simulink model "MCL"  (Simulink 9.0)
settings: Solver=ode45  StartTime=0.0  StopTime=10  RelTol=1e-3  EnableMultiTasking=on
values from neighbouring files (symbols this model uses):
  Abel = 0.0047    [MCL_init.m]
  cbel = 741.22    [MCL_init.m]
  cpc = 2.15*(10^9)    (= 2150000000)    [MCL_init.m]
  ct = 25e-12    (= 2.5e-11)    [MCL_init.m]
  dbel = 1.8    [MCL_init.m]
  g = 9.81    [MCL_init.m]
  h = 1.3    [MCL_init.m]
  Jgp = 0.293*(10^-3)    (= 0.000293)    [MCL_init.m]
  Kemfvca = 35.14    [MCL_init.m]
  Kgpemf = 72.4*(10^-3)    (= 0.0724)    [MCL_init.m]
  Kvcaemf = 35.14    [MCL_init.m]
  Lgp = 1.44*(10^-3)    (= 0.00144)    [MCL_init.m]
  Lhyd = 14.92e6    (= 14920000)    [MCL_init.m]
  Lvca = 2.9*1.0E-03    (= 0.0029)    [MCL_init.m]
  M32LMIN = 1.0E03*60    (= 60000)    [MCL_init.m]
  mbel = 1.1    [MCL_init.m]
  Mlgp = lgp*(ra^2 - ri^2)    (= 3.625e-06)    [MCL_init.m]
  PA2HG = 1.0/HG2PA    (= 0.00750061685073)    [MCL_init.m]
  RADS2TURNMIN = 60/(2*pi)    (= 9.54929658551)    [MCL_init.m]
  Rbf = 1000000000000    [MCL_init.m]
  Rgp = 0.48    [MCL_init.m]
  rhoB = 1.055E03    (= 1055)    [MCL_init.m]
  Rhyd = 572.46e6    (= 572460000)    [MCL_init.m]
  Rvca = 2.6    [MCL_init.m]
  tr0 = 44.9*(10^-6)    (= 4.49e-05)    [MCL_init.m]
  tr1 = 0.3*(10^-3)    (= 0.0003)    [MCL_init.m]
  V0 = V0comp + V0bel    (= 0.000536592894745)    [MCL_init.m]
  Vgpsv = 1.59*(10^-6)    (= 1.59e-06)    [MCL_init.m]
libraries: commnoisgen2 x5
settings Model: Creator=bahram  LastModifiedBy=lohse
settings DataIOCC: LimitDataPoints=on  SignalLoggingSaveFormat=ModelDataLogs
settings OptimizationCC: ExpressionDepthLimit=2147483647
settings DebuggingCC: SolverPrmCheckMsg=warning  MultiTaskDSMMsg=warning  MultiTaskCondExecSysMsg=none  StateNameClashWarn=warning
settings GRTTargetCC: GeneratePreprocessorConditionals=Disable all
settings ConfigComp: CovSFcnEnable=off

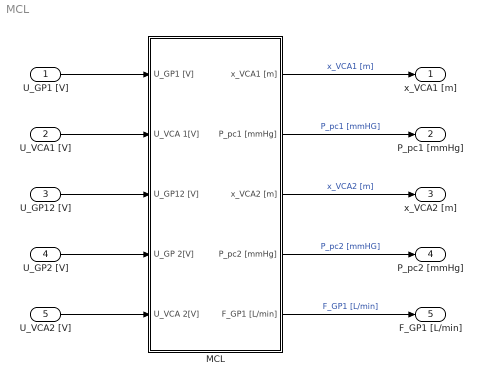
== system MCL ==
  U_GP1 [V] : Inport
  U_VCA1 [V] : Inport  Port=2
  U_GP12 [V] : Inport  Port=3
  U_GP2 [V] : Inport  Port=4
  U_VCA2 [V] : Inport  Port=5
  MCL : Subsystem
  x_VCA1 [m] : Outport
  P_pc1 [mmHg] : Outport  Port=2
  x_VCA2 [m] : Outport  Port=3
  P_pc2 [mmHg] : Outport  Port=4
  F_GP1 [L/min] : Outport  Port=5
  wires:
  MCL/1(x_VCA1 [m]) -> x_VCA1 [m]/1  "x_VCA1 [m]"
  MCL/2(P_pc1 [mmHg]) -> P_pc1 [mmHg]/1  "P_pc1 [mmHG]"
  MCL/3(x_VCA2 [m]) -> x_VCA2 [m]/1  "x_VCA2 [m]"
  MCL/4(P_pc2 [mmHg]) -> P_pc2 [mmHg]/1  "P_pc2 [mmHG]"
  U_GP1 [V]/1 -> MCL/1(U_GP1 [V])
  U_VCA1 [V]/1 -> MCL/2(U_VCA 1[V])
  U_GP12 [V]/1 -> MCL/3(U_GP12 [V])
  U_GP2 [V]/1 -> MCL/4(U_GP 2[V])
  U_VCA2 [V]/1 -> MCL/5(U_VCA 2[V])
  MCL/5(F_GP1 [L/min]) -> F_GP1 [L/min]/1  "F_GP1 [L/min]"

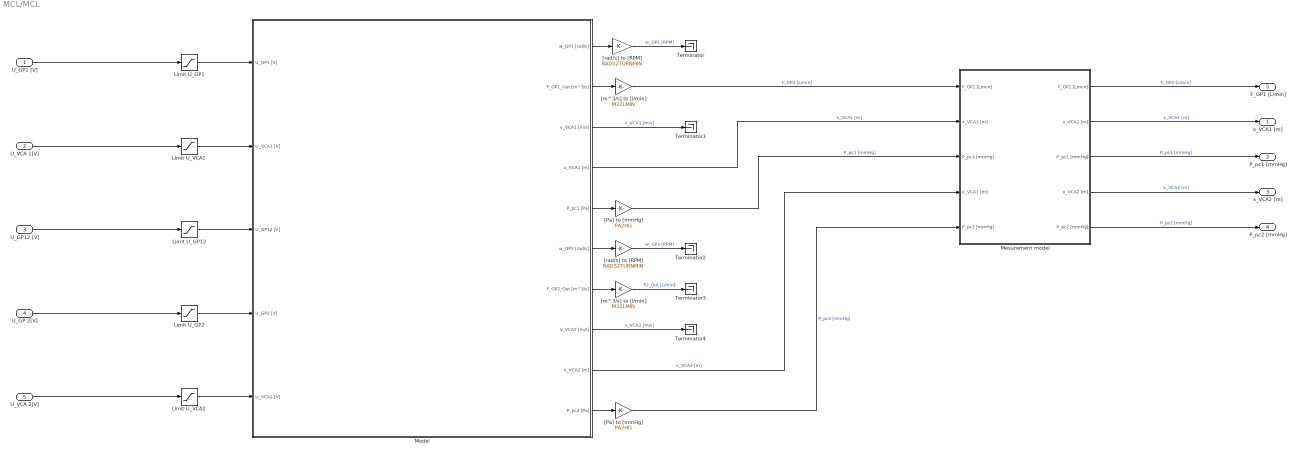
== system MCL/MCL ==
  U_GP1 [V] : Inport
  U_VCA 1[V] : Inport  Port=2
  U_GP12 [V] : Inport  Port=3
  U_GP 2[V] : Inport  Port=4
  U_VCA 2[V] : Inport  Port=5
  Limit U_GP1 : Saturate  UpperLimit=24  LowerLimit=0
  Limit U_GP12 : Saturate  UpperLimit=24  LowerLimit=0
  Limit U_GP2 : Saturate  UpperLimit=24  LowerLimit=0
  Limit U_VCA1 : Saturate  UpperLimit=24  LowerLimit=-24
  Limit U_VCA2 : Saturate  UpperLimit=24  LowerLimit=-24
  Mesurement model : Subsystem
  Model : Subsystem
  Terminator{,1..4} (5 alike) : Terminator
  "[Pa] to [mmHg] " : Gain  Gain=PA2HG
  "[Pa] to [mmHg]  " : Gain  Gain=PA2HG
  "[m^3/s] to [l/min] " : Gain  Gain=M32LMIN
  "[m^3/s] to [l/min]  " : Gain  Gain=M32LMIN
  "[rad/s] to [RPM] " : Gain  Gain=RADS2TURNMIN
  "[rad/s] to [RPM]  " : Gain  Gain=RADS2TURNMIN
  x_VCA1 [m] : Outport
  P_pc1 [mmHg] : Outport  Port=2
  x_VCA2 [m] : Outport  Port=3
  P_pc2 [mmHg] : Outport  Port=4
  F_GP1 [L/min] : Outport  Port=5
  wires:
  Model/1(w_GP1 [rad/s]) -> "[rad/s] to [RPM]  "/1
  Model/2(F_GP1_Out [m^3/s]) -> "[m^3/s] to [l/min]  "/1
  Model/5(P_pc1 [Pa]) -> "[Pa] to [mmHg] "/1
  "[rad/s] to [RPM] "/1 -> Terminator2/1  "w_GP2 [RPM]"
  Model/6(w_GP2 [rad/s]) -> "[rad/s] to [RPM] "/1
  Model/7(F_GP2_Out [m^3/s]) -> "[m^3/s] to [l/min] "/1
  Model/10(P_pc2 [Pa]) -> "[Pa] to [mmHg]  "/1
  "[m^3/s] to [l/min] "/1 -> Terminator3/1  "F2_Out [L/min]"
  Model/8(v_VCA2 [m/s]) -> Terminator4/1  "v_VCA2 [m/s]"
  Model/9(x_VCA2 [m]) -> Mesurement model/4(x_VCA2 [m])  "x_VCA2 [m]"
  "[Pa] to [mmHg]  "/1 -> Mesurement model/5(P_pc2 [mmHg])  "P_pc2 [mmHg]"
  "[rad/s] to [RPM]  "/1 -> Terminator/1  "w_GP1 [RPM]"
  "[m^3/s] to [l/min]  "/1 -> Mesurement model/1(F_GP1 [L/min])  "F_GP1 [L/min]"
  Model/3(v_VCA1 [m/s]) -> Terminator1/1  "v_VCA1 [m/s]"
  Model/4(x_VCA1 [m]) -> Mesurement model/2(x_VCA1 [m])  "x_VCA1 [m]"
  "[Pa] to [mmHg] "/1 -> Mesurement model/3(P_pc1 [mmHg])  "P_pc1 [mmHg]"
  Limit U_GP1/1 -> Model/1(U_GP1 [V])
  Limit U_GP12/1 -> Model/3(U_GP12 [V])
  Limit U_VCA1/1 -> Model/2(U_VCA1 [V])
  Limit U_VCA2/1 -> Model/5(U_VCA2 [V])
  Limit U_GP2/1 -> Model/4(U_GP2 [V])
  Mesurement model/1("F_GP1 [L/min] ") -> F_GP1 [L/min]/1  "F_GP1 [L/min]"
  Mesurement model/2("x_VCA1 [m] ") -> x_VCA1 [m]/1  "x_VCA1 [m]"
  Mesurement model/3("P_pc1 [mmHg] ") -> P_pc1 [mmHg]/1  "P_pc1 [mmHg]"
  Mesurement model/4("x_VCA2 [m] ") -> x_VCA2 [m]/1  "x_VCA2 [m]"
  Mesurement model/5("P_pc2 [mmHg] ") -> P_pc2 [mmHg]/1  "P_pc2 [mmHg]"
  U_GP1 [V]/1 -> Limit U_GP1/1
  U_VCA 1[V]/1 -> Limit U_VCA1/1
  U_GP12 [V]/1 -> Limit U_GP12/1
  U_GP 2[V]/1 -> Limit U_GP2/1
  U_VCA 2[V]/1 -> Limit U_VCA2/1

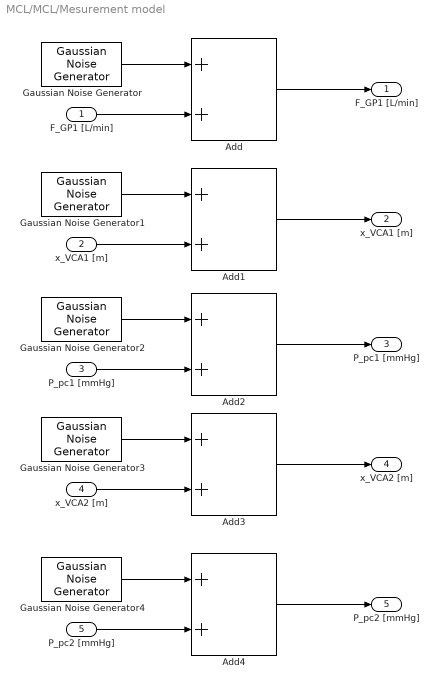
== system MCL/MCL/Mesurement model ==
  F_GP1 [L/min] : Inport
  x_VCA1 [m] : Inport  Port=2
  P_pc1 [mmHg] : Inport  Port=3
  x_VCA2 [m] : Inport  Port=4
  P_pc2 [mmHg] : Inport  Port=5
  Add{,1..4} (5 alike) : Sum
  Gaussian Noise Generator : commnoisgen2/Gaussian Noise Generator  m=0.015  d=0.01  s=100  Ts=0.001  frameBased=off  sampPerFrame=1  orient=off  outDataType=double
  Gaussian Noise Generator1 : commnoisgen2/Gaussian Noise Generator  m=0.0000003  d=0.00000002  s=200  Ts=0.001  frameBased=off  sampPerFrame=1  orient=off  outDataType=double
  Gaussian Noise Generator2 : commnoisgen2/Gaussian Noise Generator  m=0.09  d=0.002  s=115  Ts=0.001  frameBased=off  sampPerFrame=1  orient=off  outDataType=double
  Gaussian Noise Generator3 : commnoisgen2/Gaussian Noise Generator  m=0.0000001  d=0.00000001  s=300  Ts=0.001  frameBased=off  sampPerFrame=1  orient=off  outDataType=double
  Gaussian Noise Generator4 : commnoisgen2/Gaussian Noise Generator  m=0.000002  d=0.0000000015  s=230  Ts=0.001  frameBased=off  sampPerFrame=1  orient=off  outDataType=double
  "F_GP1 [L/min] " : Outport
  "x_VCA1 [m] " : Outport  Port=2
  "P_pc1 [mmHg] " : Outport  Port=3
  "x_VCA2 [m] " : Outport  Port=4
  "P_pc2 [mmHg] " : Outport  Port=5
  wires:
  P_pc1 [mmHg]/1 -> Add2/2
  x_VCA1 [m]/1 -> Add1/2
  P_pc2 [mmHg]/1 -> Add4/2
  x_VCA2 [m]/1 -> Add3/2
  Add1/1 -> "x_VCA1 [m] "/1
  Add2/1 -> "P_pc1 [mmHg] "/1
  Add3/1 -> "x_VCA2 [m] "/1
  Add4/1 -> "P_pc2 [mmHg] "/1
  Add/1 -> "F_GP1 [L/min] "/1
  Gaussian Noise Generator/1 -> Add/1
  F_GP1 [L/min]/1 -> Add/2
  Gaussian Noise Generator1/1 -> Add1/1
  Gaussian Noise Generator2/1 -> Add2/1
  Gaussian Noise Generator3/1 -> Add3/1
  Gaussian Noise Generator4/1 -> Add4/1

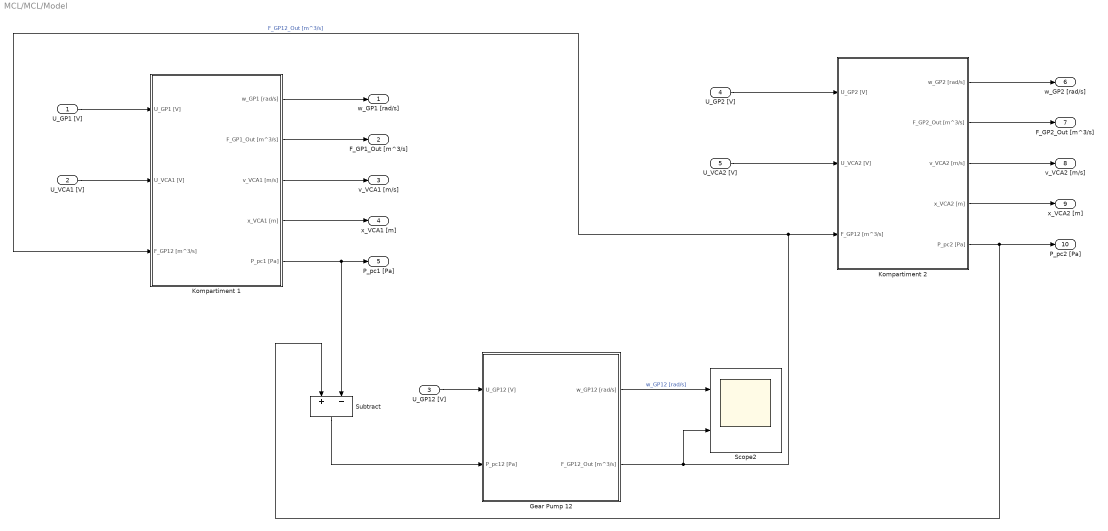
== system MCL/MCL/Model ==
  U_GP1 [V] : Inport
  U_VCA1 [V] : Inport  Port=2
  U_GP12 [V] : Inport  Port=3
  U_GP2 [V] : Inport  Port=4
  U_VCA2 [V] : Inport  Port=5
  Gear Pump 12 : Subsystem
  Kompartiment 1 : Subsystem
  Kompartiment 2 : Subsystem
  Scope2 : Scope  NumInputPorts=2
  Subtract : Sum  Inputs=+-
  w_GP1 [rad/s] : Outport
  F_GP1_Out [m^3/s] : Outport  Port=2
  v_VCA1 [m/s] : Outport  Port=3
  x_VCA1 [m] : Outport  Port=4
  P_pc1 [Pa] : Outport  Port=5
  w_GP2 [rad/s] : Outport  Port=6
  F_GP2_Out [m^3/s] : Outport  Port=7
  v_VCA2 [m/s] : Outport  Port=8
  x_VCA2 [m] : Outport  Port=9
  P_pc2 [Pa] : Outport  Port=10
  wires:
  Gear Pump 12/1(w_GP12 [rad/s]) -> Scope2/1  "w_GP12 [rad/s]"
  Kompartiment 2/1(w_GP2 [rad/s]) -> w_GP2 [rad/s]/1
  Kompartiment 2/2(F_GP2_Out [m^3/s]) -> F_GP2_Out [m^3/s]/1
  Kompartiment 2/4(x_VCA2 [m]) -> x_VCA2 [m]/1
  Kompartiment 2/3("v_VCA2 [m/s]  ") -> v_VCA2 [m/s]/1
  Kompartiment 2/5(P_pc2 [Pa]) -> P_pc2 [Pa]/1, Subtract/1
  Kompartiment 1/3("v_VCA1 [m/s]  ") -> v_VCA1 [m/s]/1
  Kompartiment 1/4(x_VCA1 [m]) -> x_VCA1 [m]/1
  Kompartiment 1/1(w_GP1 [rad/s]) -> w_GP1 [rad/s]/1
  Kompartiment 1/2(F_GP1_Out [m^3/s]) -> F_GP1_Out [m^3/s]/1
  U_GP12 [V]/1 -> Gear Pump 12/1(U_GP12 [V])
  U_GP1 [V]/1 -> Kompartiment 1/1(U_GP1 [V])
  Kompartiment 1/5(P_pc1 [Pa]) -> P_pc1 [Pa]/1, Subtract/2
  U_VCA1 [V]/1 -> Kompartiment 1/2(U_VCA1 [V])
  U_GP2 [V]/1 -> Kompartiment 2/1(U_GP2 [V])
  Subtract/1 -> Gear Pump 12/2(P_pc12 [Pa])
  U_VCA2 [V]/1 -> Kompartiment 2/2(U_VCA2 [V])
  Gear Pump 12/2(F_GP12_Out [m^3/s]) -> Scope2/2, Kompartiment 2/3(F_GP12 [m^3/s]), Kompartiment 1/3(F_GP12 [m^3/s])  "F_GP12_Out [m^3/s]"

== system MCL/MCL/Model/Gear Pump 12 ==
  U_GP12 [V] : Inport
  P_pc12 [Pa] : Inport  Port=2
  Gear Pump 12 ------> w_GP12 & i_GP12 : Subsystem
  Gear Pump 12 -----> F_GP12_Out : Subsystem
  w_GP12 [rad/s] : Outport
  F_GP12_Out [m^3/s] : Outport  Port=2
  wires:
  P_pc12 [Pa]/1 -> Gear Pump 12 -----> F_GP12_Out/2(P_pc12 [PA]), Gear Pump 12 ------> w_GP12 & i_GP12/2(P_pc12 [Pa])
  U_GP12 [V]/1 -> Gear Pump 12 ------> w_GP12 & i_GP12/1(U_GP12 [V])
  Gear Pump 12 ------> w_GP12 & i_GP12/1(w_GP12 [rad/s]) -> Gear Pump 12 -----> F_GP12_Out/1(w_GP12 [rad/s]), w_GP12 [rad/s]/1
  Gear Pump 12 -----> F_GP12_Out/1(F_GP12_Out [m^3/s]) -> F_GP12_Out [m^3/s]/1

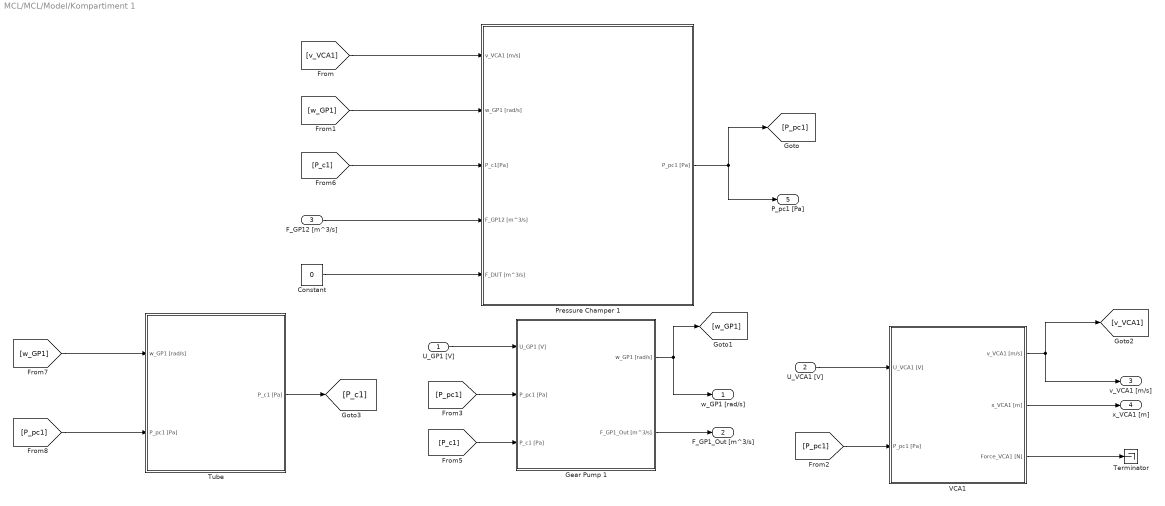
== system MCL/MCL/Model/Kompartiment 1 ==
  U_GP1 [V] : Inport
  U_VCA1 [V] : Inport  Port=2
  F_GP12 [m^3/s] : Inport  Port=3
  Constant : Constant  Value=0
  Gear Pump 1 : Subsystem
  Pressure Champer 1 : Subsystem
  Terminator : Terminator
  Tube : Subsystem
  VCA1 : Subsystem
  w_GP1 [rad/s] : Outport
  F_GP1_Out [m^3/s] : Outport  Port=2
  "v_VCA1 [m/s]  " : Outport  Port=3
  x_VCA1 [m] : Outport  Port=4
  P_pc1 [Pa] : Outport  Port=5
  wires:
  [w_GP1] -> Pressure Champer 1/2(w_GP1 [rad/s])
  U_VCA1 [V]/1 -> VCA1/1(U_VCA1 [V])
  VCA1/2(x_VCA1 [m]) -> x_VCA1 [m]/1
  VCA1/1("v_VCA1 [m/s]  ") -> "v_VCA1 [m/s]  "/1, [v_VCA1]
  Gear Pump 1/2(F_GP1_Out [m^3/s]) -> F_GP1_Out [m^3/s]/1
  Gear Pump 1/1(w_GP1 [rad/s]) -> [w_GP1], w_GP1 [rad/s]/1
  U_GP1 [V]/1 -> Gear Pump 1/1(U_GP1 [V])
  F_GP12 [m^3/s]/1 -> Pressure Champer 1/4(F_GP12 [m^3/s])
  [P_pc1] -> Gear Pump 1/2(P_pc1 [Pa])
  [v_VCA1] -> Pressure Champer 1/1(v_VCA1 [m/s])
  [P_pc1] -> Tube/2(P_pc1 [Pa])
  Tube/1(P_c1 [Pa]) -> [P_c1]
  [P_c1] -> Gear Pump 1/3(P_c1 [Pa])
  [w_GP1] -> Tube/1(w_GP1 [rad/s])
  [P_c1] -> Pressure Champer 1/3(P_c1[Pa])
  [P_pc1] -> VCA1/2("P_pc1 [Pa] ")
  Pressure Champer 1/1(P_pc1 [Pa]) -> [P_pc1], P_pc1 [Pa]/1
  Constant/1 -> Pressure Champer 1/5(F_DUT [m^3/s])
  VCA1/3(Force_VCA1 [N]) -> Terminator/1

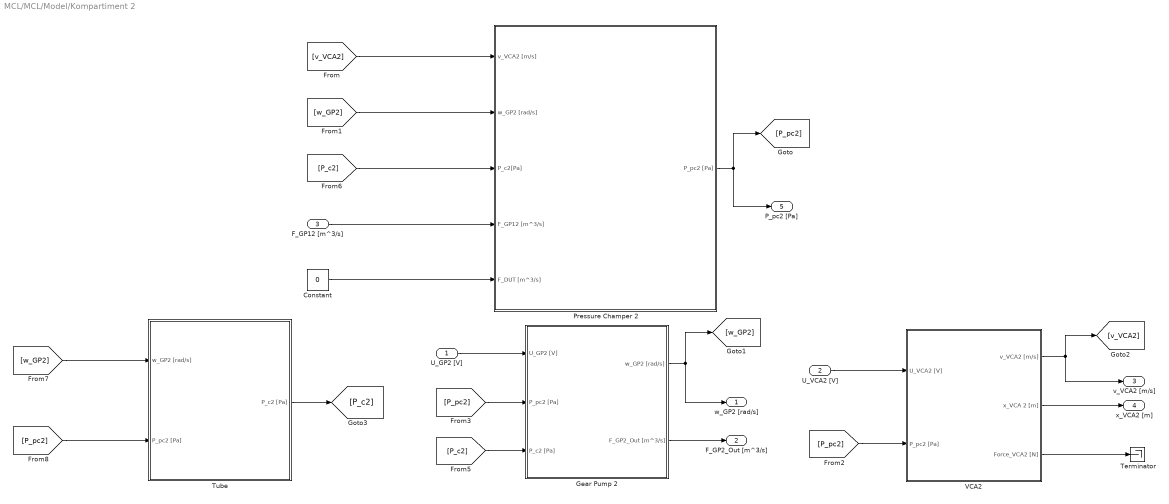
== system MCL/MCL/Model/Kompartiment 2 ==
  U_GP2 [V] : Inport
  U_VCA2 [V] : Inport  Port=2
  F_GP12 [m^3/s] : Inport  Port=3
  Constant : Constant  Value=0
  Gear Pump 2 : Subsystem
  Pressure Champer 2 : Subsystem
  Terminator : Terminator
  Tube : Subsystem
  VCA2 : Subsystem
  w_GP2 [rad/s] : Outport
  F_GP2_Out [m^3/s] : Outport  Port=2
  "v_VCA2 [m/s]  " : Outport  Port=3
  x_VCA2 [m] : Outport  Port=4
  P_pc2 [Pa] : Outport  Port=5
  wires:
  [w_GP2] -> Pressure Champer 2/2(w_GP2 [rad/s])
  U_VCA2 [V]/1 -> VCA2/1(U_VCA2 [V])
  VCA2/2(x_VCA 2 [m]) -> x_VCA2 [m]/1
  VCA2/1("v_VCA2 [m/s]  ") -> "v_VCA2 [m/s]  "/1, [v_VCA2]
  Gear Pump 2/2(F_GP2_Out [m^3/s]) -> F_GP2_Out [m^3/s]/1
  Gear Pump 2/1(w_GP2 [rad/s]) -> [w_GP2], w_GP2 [rad/s]/1
  U_GP2 [V]/1 -> Gear Pump 2/1(U_GP2 [V])
  F_GP12 [m^3/s]/1 -> Pressure Champer 2/4(F_GP12 [m^3/s])
  [P_pc2] -> Gear Pump 2/2(P_pc2 [Pa])
  [v_VCA2] -> Pressure Champer 2/1(v_VCA2 [m/s])
  [P_pc2] -> Tube/2(P_pc2 [Pa])
  Tube/1(P_c2 [Pa]) -> [P_c2]
  [P_c2] -> Gear Pump 2/3(P_c2 [Pa])
  [w_GP2] -> Tube/1(w_GP2 [rad/s])
  [P_c2] -> Pressure Champer 2/3(P_c2[Pa])
  [P_pc2] -> VCA2/2("P_pc2 [Pa] ")
  Pressure Champer 2/1(P_pc2 [Pa]) -> P_pc2 [Pa]/1, [P_pc2]
  Constant/1 -> Pressure Champer 2/5(F_DUT [m^3/s])
  VCA2/3(Force_VCA2 [N]) -> Terminator/1

== system MCL/MCL/Model/Gear Pump 12/Gear Pump 12 ------> w_GP12 & i_GP12 ==
  U_GP12 [V] : Inport
  P_pc12 [Pa] : Inport  Port=2
  Gear Pump_12 ----> i_GP12 : Subsystem
  Gear Pump_12 ----> w_GP12 : Subsystem
  Limit i_GP12 : Saturate  UpperLimit=7.5  LowerLimit=-7.5
  w_GP12 [rad/s] : Outport
  wires:
  P_pc12 [Pa]/1 -> Gear Pump_12 ----> w_GP12/2(P_pc12 [Pa])
  Gear Pump_12 ----> w_GP12/1(w_GP12 [rad/s]) -> w_GP12 [rad/s]/1, Gear Pump_12 ----> i_GP12/1(w_GP12 [rad/s])
  U_GP12 [V]/1 -> Gear Pump_12 ----> i_GP12/3(U_GP12 [V])
  Gear Pump_12 ----> i_GP12/1(i_GP12 [A]) -> Limit i_GP12/1
  Limit i_GP12/1 -> Gear Pump_12 ----> w_GP12/1(i_GP12 [A]), Gear Pump_12 ----> i_GP12/2("i_GP12 [A] ")

== system MCL/MCL/Model/Gear Pump 12/Gear Pump 12 -----> F_GP12_Out ==
  w_GP12 [rad/s] : Inport
  P_pc12 [PA] : Inport  Port=2
  Divide : Product  Inputs=*/
  Product : Product  RndMeth=Zero
  Rbf [Pa/(m^3/s)] : Constant  Value=Rbf
  Subtract1 : Sum  Inputs=+-
  Vgpsv [m^3] : Constant  Value=Vgpsv
  F_GP12_Out [m^3/s] : Outport
  wires:
  Vgpsv [m^3]/1 -> Product/2
  Subtract1/1 -> F_GP12_Out [m^3/s]/1
  P_pc12 [PA]/1 -> Divide/1
  w_GP12 [rad/s]/1 -> Product/1
  Rbf [Pa/(m^3/s)]/1 -> Divide/2
  Product/1 -> Subtract1/1
  Divide/1 -> Subtract1/2

== system MCL/MCL/Model/Kompartiment 1/Gear Pump 1 ==
  U_GP1 [V] : Inport
  P_pc1 [Pa] : Inport  Port=2
  P_c1 [Pa] : Inport  Port=3
  Gear Pump 1 ------> w_GP1 & i_GP1 : Subsystem
  Gear Pump 1 -----> F_GP1_Out : Subsystem
  w_GP1 [rad/s] : Outport
  F_GP1_Out [m^3/s] : Outport  Port=2
  wires:
  P_pc1 [Pa]/1 -> Gear Pump 1 -----> F_GP1_Out/2(P_pc1 [Pa]), Gear Pump 1 ------> w_GP1 & i_GP1/2(P_pc1 [Pa])
  U_GP1 [V]/1 -> Gear Pump 1 ------> w_GP1 & i_GP1/1(U_GP1 [V])
  P_c1 [Pa]/1 -> Gear Pump 1 -----> F_GP1_Out/3(P_c1 [Pa]), Gear Pump 1 ------> w_GP1 & i_GP1/3(P_c1 [Pa])
  Gear Pump 1 ------> w_GP1 & i_GP1/1(w_GP1 [rad/s]) -> w_GP1 [rad/s]/1, Gear Pump 1 -----> F_GP1_Out/1(w_GP1 [rad/s])
  Gear Pump 1 -----> F_GP1_Out/1(F_GP1_Out [m^3/s]) -> F_GP1_Out [m^3/s]/1

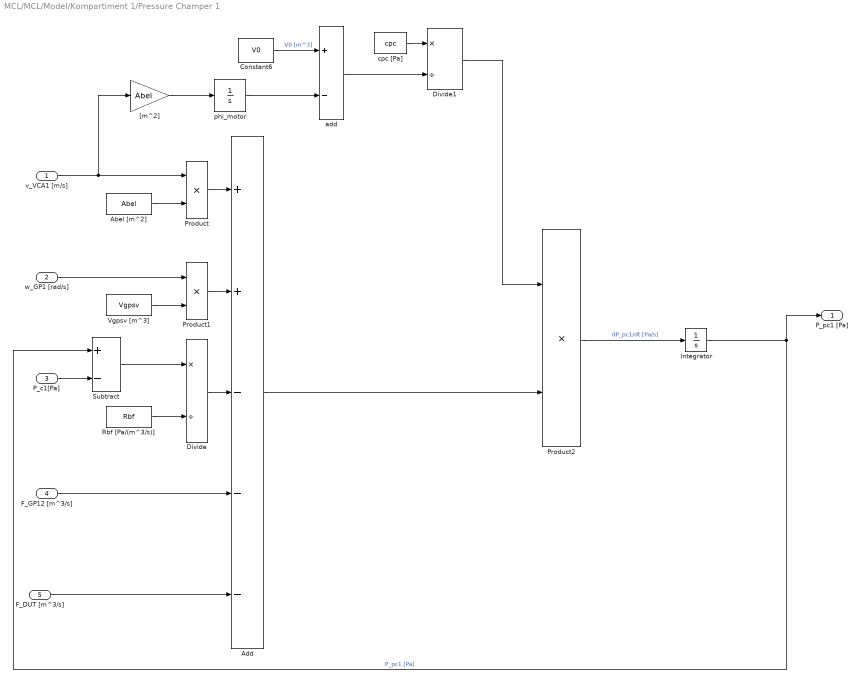
== system MCL/MCL/Model/Kompartiment 1/Pressure Champer 1 ==
  v_VCA1 [m/s] : Inport
  w_GP1 [rad/s] : Inport  Port=2
  P_c1[Pa] : Inport  Port=3
  F_GP12 [m^3/s] : Inport  Port=4
  F_DUT [m^3/s] : Inport  Port=5
  Abel [m^2] : Constant  Value=Abel
  Add : Sum  Inputs=++---
  Constant6 : Constant  Value=V0
  Divide : Product  Inputs=*/
  Divide1 : Product  Inputs=*/
  Integrator : Integrator
  Product : Product  RndMeth=Zero
  Product1 : Product  RndMeth=Zero
  Product2 : Product  RndMeth=Zero
  Rbf [Pa/(m^3/s)] : Constant  Value=Rbf
  Subtract : Sum  Inputs=+-
  Vgpsv [m^3] : Constant  Value=Vgpsv
  "[m^2]" : Gain  Gain=Abel
  add : Sum  Inputs=+-
  cpc [Pa] : Constant  Value=cpc
  phi_motor : Integrator
  P_pc1 [Pa] : Outport
  wires:
  Abel [m^2]/1 -> Product/2
  Subtract/1 -> Divide/1
  P_c1[Pa]/1 -> Subtract/2
  Rbf [Pa/(m^3/s)]/1 -> Divide/2
  Product1/1 -> Add/2
  Product/1 -> Add/1
  Divide/1 -> Add/3
  F_GP12 [m^3/s]/1 -> Add/4
  cpc [Pa]/1 -> Divide1/1
  Divide1/1 -> Product2/1
  Vgpsv [m^3]/1 -> Product1/2
  w_GP1 [rad/s]/1 -> Product1/1
  v_VCA1 [m/s]/1 -> "[m^2]"/1, Product/1
  Integrator/1 -> P_pc1 [Pa]/1, Subtract/1  "P_pc1 [Pa]"
  Add/1 -> Product2/2
  Constant6/1 -> add/1  "V0 [m^3]"
  "[m^2]"/1 -> phi_motor/1
  add/1 -> Divide1/2
  phi_motor/1 -> add/2
  Product2/1 -> Integrator/1  "dP_pc1/dt [Pa/s]"
  F_DUT [m^3/s]/1 -> Add/5

== system MCL/MCL/Model/Kompartiment 1/Tube ==
  w_GP1 [rad/s] : Inport
  P_pc1 [Pa] : Inport  Port=2
  Tube ----> F_hydr1 : Subsystem
  Tube ----> P_c1 : Subsystem
  P_c1 [Pa] : Outport
  wires:
  w_GP1 [rad/s]/1 -> Tube ----> P_c1/2(w_GP1 [rad/s])
  P_pc1 [Pa]/1 -> Tube ----> P_c1/3(P_pc1 [Pa])
  Tube ----> F_hydr1/1(F_hydr1 [m^3/s]) -> Tube ----> P_c1/1(F_hydr1 [m^3/s])
  Tube ----> P_c1/1(P_c1 [Pa]) -> P_c1 [Pa]/1, Tube ----> F_hydr1/1(" P_c1 [Pa] ")

== system MCL/MCL/Model/Kompartiment 1/VCA1 ==
  U_VCA1 [V] : Inport
  "P_pc1 [Pa] " : Inport  Port=2
  Force(X_VCA) / I_VCA [N/A] : Fcn  Expr=(-6.308*10^4)*u^2+(4.33*10^(-14))*u+35.2
  Limit i_VCA1 : Saturate  UpperLimit=7.5  LowerLimit=-7.5
  Limit x_VCA1 : Saturate  UpperLimit=0.0127  LowerLimit=-0.0127
  MATLAB Function : MATLAB Function  TreatAsAtomicUnit=on
  Product : Product  RndMeth=Zero
  Product4 : Product  RndMeth=Zero
  VCA 1-----> v_VCA1 & x_VCA1 : Subsystem
  VCA1 -----> i_VCA1 : Subsystem
  "v_VCA1 [m/s]  " : Outport
  x_VCA1 [m] : Outport  Port=2
  Force_VCA1 [N] : Outport  Port=3
  wires:
  VCA 1-----> v_VCA1 & x_VCA1/1("v_VCA1 [m/s]  ") -> Product/1, VCA1 -----> i_VCA1/2(v_VCA1 [m/s]), VCA 1-----> v_VCA1 & x_VCA1/3("v_VCA1 [m/s] ")
  VCA1 -----> i_VCA1/1("i_VCA1 [A] ") -> Limit i_VCA1/1  "i_VCA1 [A]"
  U_VCA1 [V]/1 -> VCA1 -----> i_VCA1/3(U_VCA1 [V])
  "P_pc1 [Pa] "/1 -> VCA 1-----> v_VCA1 & x_VCA1/4("P_pc1 [Pa] ")
  VCA 1-----> v_VCA1 & x_VCA1/2(x_VCA 1 [m]) -> Limit x_VCA1/1
  Limit i_VCA1/1 -> VCA1 -----> i_VCA1/1(i_VCA1 [A]), VCA 1-----> v_VCA1 & x_VCA1/1(i_VCA1 [A]), Product4/2
  Limit x_VCA1/1 -> x_VCA1 [m]/1, MATLAB Function/1(u), Force(X_VCA) / I_VCA [N/A]/1, VCA 1-----> v_VCA1 & x_VCA1/2(x_VCA1 [m])
  Force(X_VCA) / I_VCA [N/A]/1 -> Product4/1
  Product4/1 -> Force_VCA1 [N]/1  "Force_VCA1 [N]"
  MATLAB Function/1(y) -> Product/2
  Product/1 -> "v_VCA1 [m/s]  "/1

== system MCL/MCL/Model/Kompartiment 2/Gear Pump 2 ==
  U_GP2 [V] : Inport
  P_pc2 [Pa] : Inport  Port=2
  P_c2 [Pa] : Inport  Port=3
  Gear Pump 2 ------> w_GP2 & i_GP2 : Subsystem
  Gear Pump 2 -----> F_GP2_Out : Subsystem
  w_GP2 [rad/s] : Outport
  F_GP2_Out [m^3/s] : Outport  Port=2
  wires:
  P_pc2 [Pa]/1 -> Gear Pump 2 -----> F_GP2_Out/2(P_pc2 [Pa]), Gear Pump 2 ------> w_GP2 & i_GP2/2(P_pc2 [Pa])
  U_GP2 [V]/1 -> Gear Pump 2 ------> w_GP2 & i_GP2/1(U_GP2 [V])
  P_c2 [Pa]/1 -> Gear Pump 2 -----> F_GP2_Out/3(P_c2 [Pa]), Gear Pump 2 ------> w_GP2 & i_GP2/3(P_c2 [Pa])
  Gear Pump 2 ------> w_GP2 & i_GP2/1(w_GP2 [rad/s]) -> w_GP2 [rad/s]/1, Gear Pump 2 -----> F_GP2_Out/1(w_GP2 [rad/s])
  Gear Pump 2 -----> F_GP2_Out/1(F_GP2_Out [m^3/s]) -> F_GP2_Out [m^3/s]/1

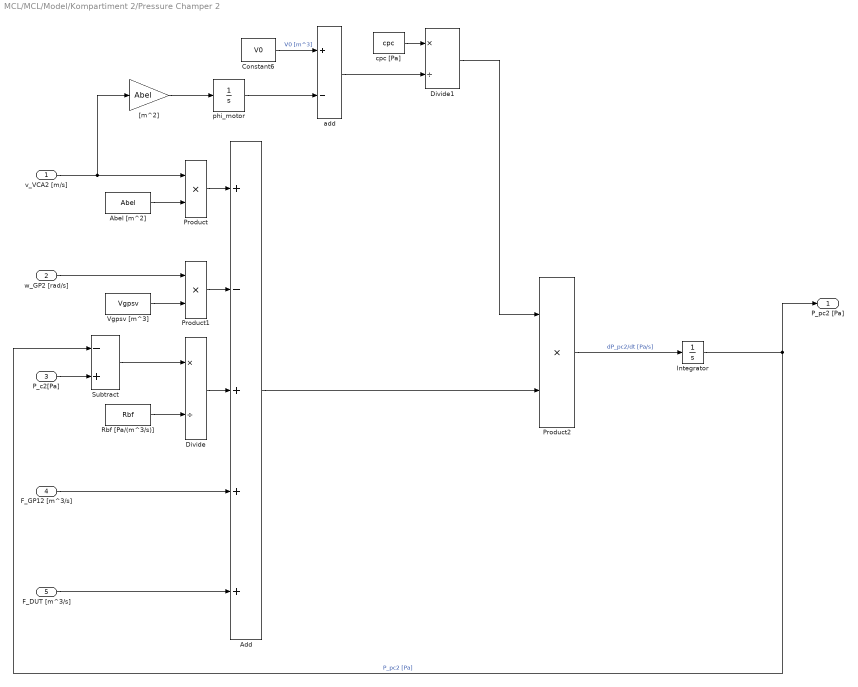
== system MCL/MCL/Model/Kompartiment 2/Pressure Champer 2 ==
  v_VCA2 [m/s] : Inport
  w_GP2 [rad/s] : Inport  Port=2
  P_c2[Pa] : Inport  Port=3
  F_GP12 [m^3/s] : Inport  Port=4
  F_DUT [m^3/s] : Inport  Port=5
  Abel [m^2] : Constant  Value=Abel
  Add : Sum  Inputs=+-+++
  Constant6 : Constant  Value=V0
  Divide : Product  Inputs=*/
  Divide1 : Product  Inputs=*/
  Integrator : Integrator
  Product : Product  RndMeth=Zero
  Product1 : Product  RndMeth=Zero
  Product2 : Product  RndMeth=Zero
  Rbf [Pa/(m^3/s)] : Constant  Value=Rbf
  Subtract : Sum  Inputs=-+
  Vgpsv [m^3] : Constant  Value=Vgpsv
  "[m^2]" : Gain  Gain=Abel
  add : Sum  Inputs=+-
  cpc [Pa] : Constant  Value=cpc
  phi_motor : Integrator
  P_pc2 [Pa] : Outport
  wires:
  Abel [m^2]/1 -> Product/2
  Subtract/1 -> Divide/1
  P_c2[Pa]/1 -> Subtract/2
  Rbf [Pa/(m^3/s)]/1 -> Divide/2
  Product1/1 -> Add/2
  Product/1 -> Add/1
  Divide/1 -> Add/3
  F_GP12 [m^3/s]/1 -> Add/4
  cpc [Pa]/1 -> Divide1/1
  Divide1/1 -> Product2/1
  Vgpsv [m^3]/1 -> Product1/2
  w_GP2 [rad/s]/1 -> Product1/1
  v_VCA2 [m/s]/1 -> "[m^2]"/1, Product/1
  Integrator/1 -> P_pc2 [Pa]/1, Subtract/1  "P_pc2 [Pa]"
  Add/1 -> Product2/2
  Constant6/1 -> add/1  "V0 [m^3]"
  "[m^2]"/1 -> phi_motor/1
  add/1 -> Divide1/2
  phi_motor/1 -> add/2
  Product2/1 -> Integrator/1  "dP_pc2/dt [Pa/s]"
  F_DUT [m^3/s]/1 -> Add/5

== system MCL/MCL/Model/Kompartiment 2/Tube ==
  w_GP2 [rad/s] : Inport
  P_pc2 [Pa] : Inport  Port=2
  Tube ----> F_hydr2 : Subsystem
  Tube ----> P_c2 : Subsystem
  P_c2 [Pa] : Outport
  wires:
  w_GP2 [rad/s]/1 -> Tube ----> P_c2/2(w_GP2 [rad/s])
  P_pc2 [Pa]/1 -> Tube ----> P_c2/3(P_pc2 [Pa])
  Tube ----> F_hydr2/1(F_hydr2 [m^3/s]) -> Tube ----> P_c2/1(F_hydr2 [m^3/s])
  Tube ----> P_c2/1(P_c2 [Pa]) -> P_c2 [Pa]/1, Tube ----> F_hydr2/1(" P_c2 [Pa] ")

== system MCL/MCL/Model/Kompartiment 2/VCA2 ==
  U_VCA2 [V] : Inport
  "P_pc2 [Pa] " : Inport  Port=2
  Force(X_VCA) / I_VCA [N/A] : Fcn  Expr=(-6.308*10^4)*u^2+(4.33*10^(-14))*u+35.2
  Limit i_VCA2 : Saturate  UpperLimit=7.5  LowerLimit=-7.5
  Limit x_VCA2 : Saturate  UpperLimit=0.0127  LowerLimit=-0.0127
  MATLAB Function1 : MATLAB Function  TreatAsAtomicUnit=on
  Product1 : Product  RndMeth=Zero
  Product4 : Product  RndMeth=Zero
  VCA 2-----> v_VCA2 & x_VCA2 : Subsystem
  VCA2 -----> i_VCA2 : Subsystem
  "v_VCA2 [m/s]  " : Outport
  x_VCA 2 [m] : Outport  Port=2
  Force_VCA2 [N] : Outport  Port=3
  wires:
  VCA 2-----> v_VCA2 & x_VCA2/1("v_VCA2 [m/s]  ") -> Product1/1, VCA2 -----> i_VCA2/2(v_VCA2 [m/s]), VCA 2-----> v_VCA2 & x_VCA2/3("v_VCA2 [m/s] ")
  VCA2 -----> i_VCA2/1("i_VCA2 [A] ") -> Limit i_VCA2/1  "i_VCA2 [A]"
  U_VCA2 [V]/1 -> VCA2 -----> i_VCA2/3(U_VCA2 [V])
  "P_pc2 [Pa] "/1 -> VCA 2-----> v_VCA2 & x_VCA2/4("P_pc2 [Pa] ")
  VCA 2-----> v_VCA2 & x_VCA2/2(x_VCA 2 [m]) -> Limit x_VCA2/1
  Limit i_VCA2/1 -> VCA2 -----> i_VCA2/1(i_VCA2 [A]), VCA 2-----> v_VCA2 & x_VCA2/1(i_VCA2 [A]), Product4/2
  Limit x_VCA2/1 -> MATLAB Function1/1(u), x_VCA 2 [m]/1, Force(X_VCA) / I_VCA [N/A]/1, VCA 2-----> v_VCA2 & x_VCA2/2(x_VCA2 [m])
  Force(X_VCA) / I_VCA [N/A]/1 -> Product4/1
  Product4/1 -> Force_VCA2 [N]/1  "Force_VCA2 [N]"
  MATLAB Function1/1(y) -> Product1/2
  Product1/1 -> "v_VCA2 [m/s]  "/1

== system MCL/MCL/Model/Gear Pump 12/Gear Pump 12 ------> w_GP12 & i_GP12/Gear Pump_12 ----> i_GP12 ==
  w_GP12 [rad/s] : Inport
  "i_GP12 [A] " : Inport  Port=2
  U_GP12 [V] : Inport  Port=3
  Add : Sum  Inputs=--+
  Divide : Product  Inputs=*/
  Integrator : Integrator
  Kgpemf [Vs] : Constant  Value=Kgpemf
  Lgp [H] : Constant  Value=Lgp
  Product : Product  RndMeth=Zero
  Product1 : Product  RndMeth=Zero
  Rgp [Ohm] : Constant  Value=Rgp
  i_GP12 [A] : Outport
  wires:
  w_GP12 [rad/s]/1 -> Product/1
  Kgpemf [Vs]/1 -> Product/2
  "i_GP12 [A] "/1 -> Product1/1
  Rgp [Ohm]/1 -> Product1/2
  Product1/1 -> Add/2
  Product/1 -> Add/1
  U_GP12 [V]/1 -> Add/3
  Lgp [H]/1 -> Divide/2
  Divide/1 -> Integrator/1  "di_GP12/dt [A/s]"
  Add/1 -> Divide/1
  Integrator/1 -> i_GP12 [A]/1  "i_GP12[A]"

== system MCL/MCL/Model/Gear Pump 12/Gear Pump 12 ------> w_GP12 & i_GP12/Gear Pump_12 ----> w_GP12 ==
  i_GP12 [A] : Inport
  P_pc12 [Pa] : Inport  Port=2
  Constant : Constant  Value=tr0
  Constant1 : Constant  Value=tr1
  Divide : Product  Inputs=*/
  Integrator : Integrator
  Kgpemf [Vs] : Constant  Value=Kgpemf
  Mlgp [m^3] : Constant  Value=Mlgp
  Product{,1..3} (4 alike) : Product  RndMeth=Zero
  Sign : Signum  ZeroCross=off
  Subtract1 : Sum  Inputs=+---
  jgp [kgm^2] : Constant  Value=Jgp
  w_GP12 [rad/s] : Outport
  wires:
  Subtract1/1 -> Divide/1
  jgp [kgm^2]/1 -> Divide/2
  Integrator/1 -> Product3/1, Sign/1, w_GP12 [rad/s]/1  "w_GP12[rad/s]"
  Divide/1 -> Integrator/1  "dw_GP12/dt [rad/s^2]"
  i_GP12 [A]/1 -> Product/1
  Kgpemf [Vs]/1 -> Product/2
  Product/1 -> Subtract1/1
  Product1/1 -> Subtract1/2
  P_pc12 [Pa]/1 -> Product1/1
  Mlgp [m^3]/1 -> Product1/2
  Sign/1 -> Product2/1
  Constant/1 -> Product2/2
  Product3/1 -> Subtract1/4
  Constant1/1 -> Product3/2
  Product2/1 -> Subtract1/3

== system MCL/MCL/Model/Kompartiment 1/Gear Pump 1/Gear Pump 1 ------> w_GP1 & i_GP1 ==
  U_GP1 [V] : Inport
  P_pc1 [Pa] : Inport  Port=2
  P_c1 [Pa] : Inport  Port=3
  "Gear Pump_1 ----> i_GP1 " : Subsystem
  Gear Pump_1 ----> w_GP1 : Subsystem
  Limit i_GP1 : Saturate  UpperLimit=7.5  LowerLimit=-7.5
  w_GP1 [rad/s] : Outport
  wires:
  P_c1 [Pa]/1 -> Gear Pump_1 ----> w_GP1/3(P_c1 [Pa])
  P_pc1 [Pa]/1 -> Gear Pump_1 ----> w_GP1/2(P_pc1 [Pa])
  Gear Pump_1 ----> w_GP1/1(w_GP1 [rad/s]) -> w_GP1 [rad/s]/1, "Gear Pump_1 ----> i_GP1 "/1(w_GP1 [rad/s])
  U_GP1 [V]/1 -> "Gear Pump_1 ----> i_GP1 "/3(U_GP1 [V])
  "Gear Pump_1 ----> i_GP1 "/1(i_GP1 [A]) -> Limit i_GP1/1
  Limit i_GP1/1 -> Gear Pump_1 ----> w_GP1/1(i_GP1 [A]), "Gear Pump_1 ----> i_GP1 "/2("i_GP1 [A] ")

== system MCL/MCL/Model/Kompartiment 1/Gear Pump 1/Gear Pump 1 -----> F_GP1_Out ==
  w_GP1 [rad/s] : Inport
  P_pc1 [Pa] : Inport  Port=2
  P_c1 [Pa] : Inport  Port=3
  Divide : Product  Inputs=*/
  Product : Product  RndMeth=Zero
  Rbf [Pa/(m^3/s)] : Constant  Value=Rbf
  Subtract : Sum  Inputs=+-
  Subtract1 : Sum  Inputs=+-
  Vgpsv [m^3] : Constant  Value=Vgpsv
  F_GP1_Out [m^3/s] : Outport
  wires:
  Vgpsv [m^3]/1 -> Product/2
  Subtract1/1 -> F_GP1_Out [m^3/s]/1
  Subtract/1 -> Divide/1
  w_GP1 [rad/s]/1 -> Product/1
  P_pc1 [Pa]/1 -> Subtract/1
  P_c1 [Pa]/1 -> Subtract/2
  Rbf [Pa/(m^3/s)]/1 -> Divide/2
  Product/1 -> Subtract1/1
  Divide/1 -> Subtract1/2

== system MCL/MCL/Model/Kompartiment 1/Tube/Tube ----> F_hydr1 ==
  " P_c1 [Pa] " : Inport
  Add : Sum  Inputs=--+
  Divide : Product  Inputs=*/
  Integrator : Integrator
  Lhyd [kg/m^4] : Constant  Value=Lhyd
  Product : Product  RndMeth=Zero
  Rhyd [Pa/(m^3/s)] : Constant  Value=Rhyd
  "[Pa]" : Constant  Value=rhoB*g*h
  F_hydr1 [m^3/s] : Outport
  wires:
  Integrator/1 -> F_hydr1 [m^3/s]/1, Product/1  "F_hydr1 [m^3/s]"
  " P_c1 [Pa] "/1 -> Add/1
  Product/1 -> Add/2
  Lhyd [kg/m^4]/1 -> Divide/2
  Add/1 -> Divide/1
  Divide/1 -> Integrator/1  "dF_hydr1/dt [m^3/s^2]"
  Rhyd [Pa/(m^3/s)]/1 -> Product/2
  "[Pa]"/1 -> Add/3

== system MCL/MCL/Model/Kompartiment 1/Tube/Tube ----> P_c1 ==
  F_hydr1 [m^3/s] : Inport
  w_GP1 [rad/s] : Inport  Port=2
  P_pc1 [Pa] : Inport  Port=3
  Add : Sum  Inputs=+-+
  Divide : Product  Inputs=*/
  Divide1 : Product  Inputs=*/
  Integrator : Integrator
  Product : Product  RndMeth=Zero
  Subtract : Sum  Inputs=+-
  Vgpsv [m^3] : Constant  Value=Vgpsv
  "[Pa/(m^3/s)]" : Constant  Value=Rbf
  ct [s^2*m^4/Kg] : Constant  Value=ct
  P_c1 [Pa] : Outport
  wires:
  Vgpsv [m^3]/1 -> Product/2
  w_GP1 [rad/s]/1 -> Product/1
  Subtract/1 -> Divide/1
  F_hydr1 [m^3/s]/1 -> Add/1
  P_pc1 [Pa]/1 -> Subtract/1
  "[Pa/(m^3/s)]"/1 -> Divide/2
  Product/1 -> Add/2
  Divide/1 -> Add/3
  ct [s^2*m^4/Kg]/1 -> Divide1/2
  Add/1 -> Divide1/1
  Integrator/1 -> Subtract/2, P_c1 [Pa]/1  "P_c1 [Pa]"
  Divide1/1 -> Integrator/1  "dP_c1/dt [Pa/s]"

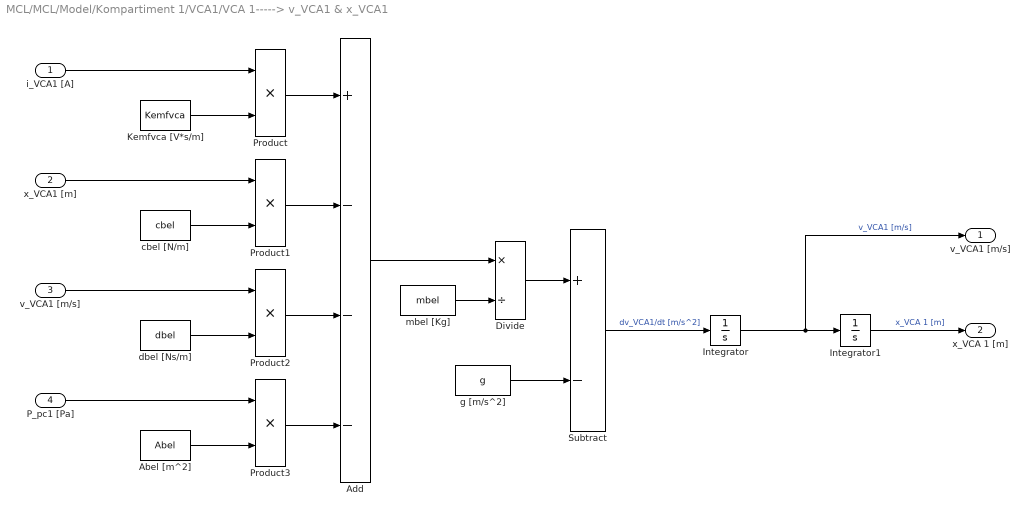
== system MCL/MCL/Model/Kompartiment 1/VCA1/VCA 1-----> v_VCA1 & x_VCA1 ==
  i_VCA1 [A] : Inport
  x_VCA1 [m] : Inport  Port=2
  "v_VCA1 [m/s] " : Inport  Port=3
  "P_pc1 [Pa] " : Inport  Port=4
  Abel [m^2] : Constant  Value=Abel
  Add : Sum  Inputs=+---
  Divide : Product  Inputs=*/
  Integrator : Integrator
  Integrator1 : Integrator
  Kemfvca [V*s/m] : Constant  Value=Kemfvca
  Product{,1..3} (4 alike) : Product  RndMeth=Zero
  Subtract : Sum  Inputs=+-
  cbel [N/m] : Constant  Value=cbel
  dbel [Ns/m] : Constant  Value=dbel
  g [m/s^2] : Constant  Value=g
  mbel [Kg] : Constant  Value=mbel
  "v_VCA1 [m/s]  " : Outport
  x_VCA 1 [m] : Outport  Port=2
  wires:
  Divide/1 -> Subtract/1
  Integrator1/1 -> x_VCA 1 [m]/1  "x_VCA 1 [m]"
  dbel [Ns/m]/1 -> Product2/2
  Kemfvca [V*s/m]/1 -> Product/2
  Add/1 -> Divide/1
  cbel [N/m]/1 -> Product1/2
  Product/1 -> Add/1
  "v_VCA1 [m/s] "/1 -> Product2/1
  i_VCA1 [A]/1 -> Product/1
  x_VCA1 [m]/1 -> Product1/1
  Product1/1 -> Add/2
  Subtract/1 -> Integrator/1  "dv_VCA1/dt [m/s^2]"
  g [m/s^2]/1 -> Subtract/2
  Product2/1 -> Add/3
  Product3/1 -> Add/4
  Abel [m^2]/1 -> Product3/2
  "P_pc1 [Pa] "/1 -> Product3/1
  mbel [Kg]/1 -> Divide/2
  Integrator/1 -> "v_VCA1 [m/s]  "/1, Integrator1/1  "v_VCA1 [m/s]"

== system MCL/MCL/Model/Kompartiment 1/VCA1/VCA1 -----> i_VCA1 ==
  i_VCA1 [A] : Inport
  v_VCA1 [m/s] : Inport  Port=2
  U_VCA1 [V] : Inport  Port=3
  Add : Sum  Inputs=--+
  Divide : Product  Inputs=*/
  Integrator : Integrator
  Kvcaemf [N/A] : Constant  Value=Kvcaemf
  Lvca [H] : Constant  Value=Lvca
  Product : Product  RndMeth=Zero
  Product1 : Product  RndMeth=Zero
  Rvca [Ohm] : Constant  Value=Rvca
  "i_VCA1 [A] " : Outport
  wires:
  Product/1 -> Add/1
  v_VCA1 [m/s]/1 -> Product1/1
  U_VCA1 [V]/1 -> Add/3
  i_VCA1 [A]/1 -> Product/1
  Rvca [Ohm]/1 -> Product/2
  Product1/1 -> Add/2
  Kvcaemf [N/A]/1 -> Product1/2
  Divide/1 -> Integrator/1  "di_VCA1/dt[A/s]"
  Lvca [H]/1 -> Divide/2
  Integrator/1 -> "i_VCA1 [A] "/1  "i_VCA1 [A]"
  Add/1 -> Divide/1

== system MCL/MCL/Model/Kompartiment 2/Gear Pump 2/Gear Pump 2 ------> w_GP2 & i_GP2 ==
  U_GP2 [V] : Inport
  P_pc2 [Pa] : Inport  Port=2
  P_c2 [Pa] : Inport  Port=3
  "Gear Pump 2 ----> i_GP2 " : Subsystem
  Gear Pump 2 ----> w_GP2 : Subsystem
  Limit i_GP2 : Saturate  UpperLimit=7.5  LowerLimit=-7.5
  w_GP2 [rad/s] : Outport
  wires:
  P_c2 [Pa]/1 -> Gear Pump 2 ----> w_GP2/3(P_c2 [Pa])
  P_pc2 [Pa]/1 -> Gear Pump 2 ----> w_GP2/2(P_pc2 [Pa])
  Gear Pump 2 ----> w_GP2/1(w_GP2 [rad/s]) -> w_GP2 [rad/s]/1, "Gear Pump 2 ----> i_GP2 "/1(w_GP2 [rad/s])
  U_GP2 [V]/1 -> "Gear Pump 2 ----> i_GP2 "/3(U_GP2 [V])
  "Gear Pump 2 ----> i_GP2 "/1(i_GP2 [A]) -> Limit i_GP2/1
  Limit i_GP2/1 -> Gear Pump 2 ----> w_GP2/1(i_GP2 [A]), "Gear Pump 2 ----> i_GP2 "/2("i_GP2 [A] ")

== system MCL/MCL/Model/Kompartiment 2/Gear Pump 2/Gear Pump 2 -----> F_GP2_Out ==
  w_GP2 [rad/s] : Inport
  P_pc2 [Pa] : Inport  Port=2
  P_c2 [Pa] : Inport  Port=3
  Divide : Product  Inputs=*/
  Product : Product  RndMeth=Zero
  Rbf [Pa/(m^3/s)] : Constant  Value=Rbf
  Subtract : Sum  Inputs=-+
  Subtract1 : Sum  Inputs=+-
  Vgpsv [m^3] : Constant  Value=Vgpsv
  F_GP2_Out [m^3/s] : Outport
  wires:
  Vgpsv [m^3]/1 -> Product/2
  Subtract1/1 -> F_GP2_Out [m^3/s]/1
  Subtract/1 -> Divide/1
  w_GP2 [rad/s]/1 -> Product/1
  P_pc2 [Pa]/1 -> Subtract/1
  P_c2 [Pa]/1 -> Subtract/2
  Rbf [Pa/(m^3/s)]/1 -> Divide/2
  Product/1 -> Subtract1/1
  Divide/1 -> Subtract1/2

== system MCL/MCL/Model/Kompartiment 2/Tube/Tube ----> F_hydr2 ==
  " P_c2 [Pa] " : Inport
  Add : Sum  Inputs=---
  Divide : Product  Inputs=*/
  Integrator : Integrator
  Lhyd [kg/m^4] : Constant  Value=Lhyd
  Product : Product  RndMeth=Zero
  Rhyd [Pa/(m^3/s)] : Constant  Value=Rhyd
  "[N/m^2]" : Constant  Value=rhoB*g*h
  F_hydr2 [m^3/s] : Outport
  wires:
  Integrator/1 -> F_hydr2 [m^3/s]/1, Product/1  "F_hydr2 [m^3/s]"
  " P_c2 [Pa] "/1 -> Add/1
  Product/1 -> Add/2
  Lhyd [kg/m^4]/1 -> Divide/2
  Add/1 -> Divide/1
  Divide/1 -> Integrator/1  "dF_hydr2/dt [m^3/s^2]"
  Rhyd [Pa/(m^3/s)]/1 -> Product/2
  "[N/m^2]"/1 -> Add/3

== system MCL/MCL/Model/Kompartiment 2/Tube/Tube ----> P_c2 ==
  F_hydr2 [m^3/s] : Inport
  w_GP2 [rad/s] : Inport  Port=2
  P_pc2 [Pa] : Inport  Port=3
  Add : Sum  Inputs=+-+
  Divide : Product  Inputs=*/
  Divide1 : Product  Inputs=*/
  Integrator : Integrator
  Product : Product  RndMeth=Zero
  Subtract : Sum  Inputs=+-
  Vgpsv [m^3] : Constant  Value=Vgpsv
  "[Pa/(m^3/s)]" : Constant  Value=Rbf
  ct [s^2*m^4/Kg] : Constant  Value=ct
  P_c2 [Pa] : Outport
  wires:
  Vgpsv [m^3]/1 -> Product/2
  w_GP2 [rad/s]/1 -> Product/1
  Subtract/1 -> Divide/1
  F_hydr2 [m^3/s]/1 -> Add/1
  P_pc2 [Pa]/1 -> Subtract/1
  "[Pa/(m^3/s)]"/1 -> Divide/2
  Product/1 -> Add/2
  Divide/1 -> Add/3
  ct [s^2*m^4/Kg]/1 -> Divide1/2
  Add/1 -> Divide1/1
  Integrator/1 -> Subtract/2, P_c2 [Pa]/1  "P_c2 [Pa]"
  Divide1/1 -> Integrator/1  "dP_c2/dt [Pa/s]"

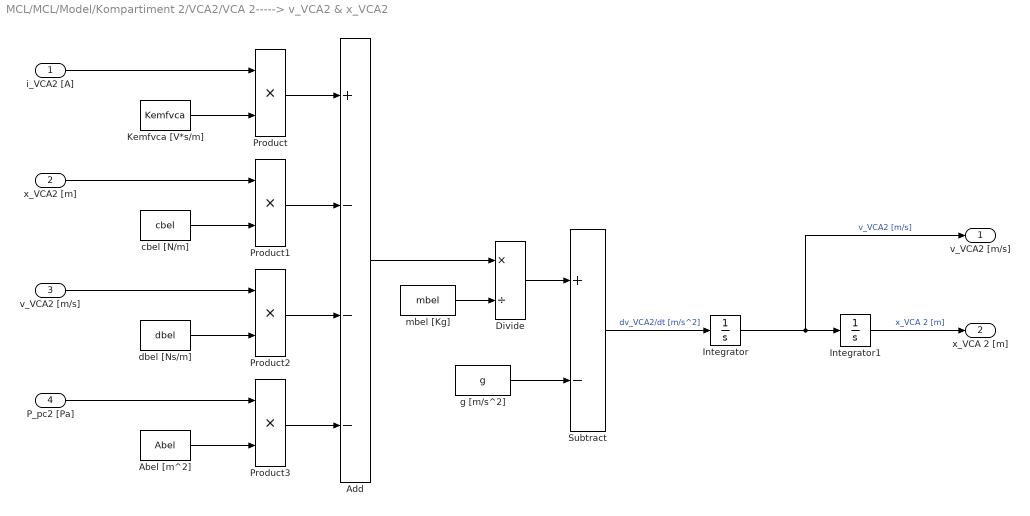
== system MCL/MCL/Model/Kompartiment 2/VCA2/VCA 2-----> v_VCA2 & x_VCA2 ==
  i_VCA2 [A] : Inport
  x_VCA2 [m] : Inport  Port=2
  "v_VCA2 [m/s] " : Inport  Port=3
  "P_pc2 [Pa] " : Inport  Port=4
  Abel [m^2] : Constant  Value=Abel
  Add : Sum  Inputs=+---
  Divide : Product  Inputs=*/
  Integrator : Integrator
  Integrator1 : Integrator
  Kemfvca [V*s/m] : Constant  Value=Kemfvca
  Product{,1..3} (4 alike) : Product  RndMeth=Zero
  Subtract : Sum  Inputs=+-
  cbel [N/m] : Constant  Value=cbel
  dbel [Ns/m] : Constant  Value=dbel
  g [m/s^2] : Constant  Value=g
  mbel [Kg] : Constant  Value=mbel
  "v_VCA2 [m/s]  " : Outport
  x_VCA 2 [m] : Outport  Port=2
  wires:
  Divide/1 -> Subtract/1
  Integrator1/1 -> x_VCA 2 [m]/1  "x_VCA 2 [m]"
  dbel [Ns/m]/1 -> Product2/2
  Kemfvca [V*s/m]/1 -> Product/2
  Add/1 -> Divide/1
  cbel [N/m]/1 -> Product1/2
  Product/1 -> Add/1
  "v_VCA2 [m/s] "/1 -> Product2/1
  i_VCA2 [A]/1 -> Product/1
  x_VCA2 [m]/1 -> Product1/1
  Product1/1 -> Add/2
  Subtract/1 -> Integrator/1  "dv_VCA2/dt [m/s^2]"
  g [m/s^2]/1 -> Subtract/2
  Product2/1 -> Add/3
  Product3/1 -> Add/4
  Abel [m^2]/1 -> Product3/2
  "P_pc2 [Pa] "/1 -> Product3/1
  mbel [Kg]/1 -> Divide/2
  Integrator/1 -> "v_VCA2 [m/s]  "/1, Integrator1/1  "v_VCA2 [m/s]"

== system MCL/MCL/Model/Kompartiment 2/VCA2/VCA2 -----> i_VCA2 ==
  i_VCA2 [A] : Inport
  v_VCA2 [m/s] : Inport  Port=2
  U_VCA2 [V] : Inport  Port=3
  Add : Sum  Inputs=--+
  Divide : Product  Inputs=*/
  Integrator : Integrator
  Kvcaemf [N/A] : Constant  Value=Kvcaemf
  Lvca [H] : Constant  Value=Lvca
  Product : Product  RndMeth=Zero
  Product1 : Product  RndMeth=Zero
  Rvca [Ohm] : Constant  Value=Rvca
  "i_VCA2 [A] " : Outport
  wires:
  Product/1 -> Add/1
  v_VCA2 [m/s]/1 -> Product1/1
  U_VCA2 [V]/1 -> Add/3
  i_VCA2 [A]/1 -> Product/1
  Rvca [Ohm]/1 -> Product/2
  Product1/1 -> Add/2
  Kvcaemf [N/A]/1 -> Product1/2
  Divide/1 -> Integrator/1  "di_VCA2/dt[A/s]"
  Lvca [H]/1 -> Divide/2
  Integrator/1 -> "i_VCA2 [A] "/1  "i_VCA2 [A]"
  Add/1 -> Divide/1

== system MCL/MCL/Model/Kompartiment 1/Gear Pump 1/Gear Pump 1 ------> w_GP1 & i_GP1/Gear Pump_1 ----> i_GP1  ==
  w_GP1 [rad/s] : Inport
  "i_GP1 [A] " : Inport  Port=2
  U_GP1 [V] : Inport  Port=3
  Add : Sum  Inputs=--+
  Divide : Product  Inputs=*/
  Integrator : Integrator
  Kgpemf [Vs] : Constant  Value=Kgpemf
  Lgp [H] : Constant  Value=Lgp
  Product : Product  RndMeth=Zero
  Product1 : Product  RndMeth=Zero
  Rgp [Ohm] : Constant  Value=Rgp
  i_GP1 [A] : Outport
  wires:
  w_GP1 [rad/s]/1 -> Product/1
  Kgpemf [Vs]/1 -> Product/2
  "i_GP1 [A] "/1 -> Product1/1
  Rgp [Ohm]/1 -> Product1/2
  Product1/1 -> Add/2
  Product/1 -> Add/1
  U_GP1 [V]/1 -> Add/3
  Lgp [H]/1 -> Divide/2
  Divide/1 -> Integrator/1  "di_GP1/dt [A/s]"
  Add/1 -> Divide/1
  Integrator/1 -> i_GP1 [A]/1  "i_GP1 [A]"

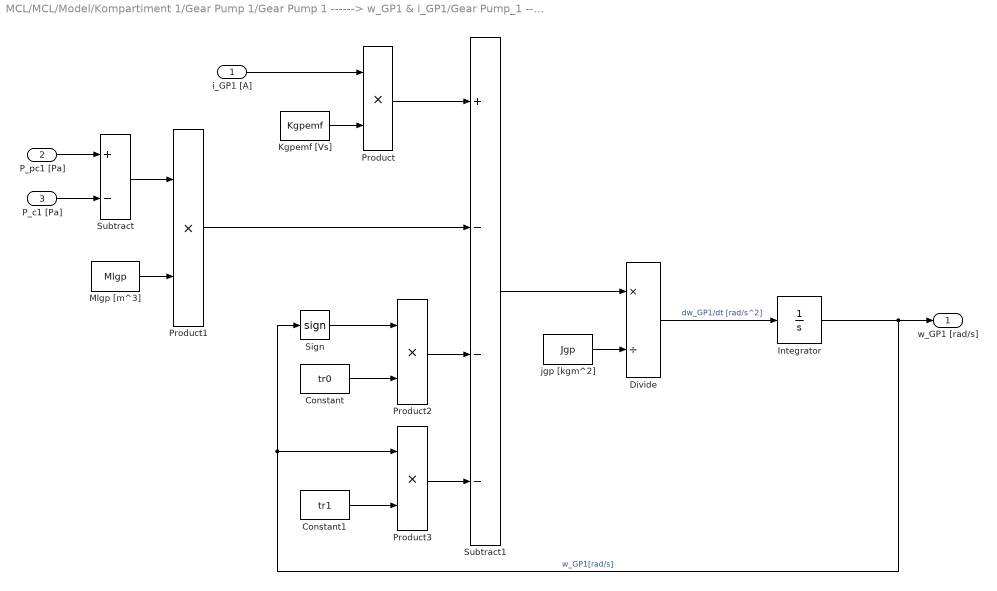
== system MCL/MCL/Model/Kompartiment 1/Gear Pump 1/Gear Pump 1 ------> w_GP1 & i_GP1/Gear Pump_1 ----> w_GP1 ==
  i_GP1 [A] : Inport
  P_pc1 [Pa] : Inport  Port=2
  P_c1 [Pa] : Inport  Port=3
  Constant : Constant  Value=tr0
  Constant1 : Constant  Value=tr1
  Divide : Product  Inputs=*/
  Integrator : Integrator
  Kgpemf [Vs] : Constant  Value=Kgpemf
  Mlgp [m^3] : Constant  Value=Mlgp
  Product{,1..3} (4 alike) : Product  RndMeth=Zero
  Sign : Signum  ZeroCross=off
  Subtract : Sum  Inputs=+-
  Subtract1 : Sum  Inputs=+---
  jgp [kgm^2] : Constant  Value=Jgp
  w_GP1 [rad/s] : Outport
  wires:
  Subtract1/1 -> Divide/1
  jgp [kgm^2]/1 -> Divide/2
  Integrator/1 -> Product3/1, Sign/1, w_GP1 [rad/s]/1  "w_GP1[rad/s]"
  Divide/1 -> Integrator/1  "dw_GP1/dt [rad/s^2]"
  i_GP1 [A]/1 -> Product/1
  Kgpemf [Vs]/1 -> Product/2
  Product/1 -> Subtract1/1
  Product1/1 -> Subtract1/2
  Subtract/1 -> Product1/1
  Mlgp [m^3]/1 -> Product1/2
  P_c1 [Pa]/1 -> Subtract/2
  P_pc1 [Pa]/1 -> Subtract/1
  Sign/1 -> Product2/1
  Constant/1 -> Product2/2
  Product3/1 -> Subtract1/4
  Constant1/1 -> Product3/2
  Product2/1 -> Subtract1/3

== system MCL/MCL/Model/Kompartiment 2/Gear Pump 2/Gear Pump 2 ------> w_GP2 & i_GP2/Gear Pump 2 ----> i_GP2  ==
  w_GP2 [rad/s] : Inport
  "i_GP2 [A] " : Inport  Port=2
  U_GP2 [V] : Inport  Port=3
  Add : Sum  Inputs=--+
  Divide : Product  Inputs=*/
  Integrator : Integrator
  Kgpemf [Vs] : Constant  Value=Kgpemf
  Lgp [H] : Constant  Value=Lgp
  Product : Product  RndMeth=Zero
  Product1 : Product  RndMeth=Zero
  Rgp [Ohm] : Constant  Value=Rgp
  i_GP2 [A] : Outport
  wires:
  w_GP2 [rad/s]/1 -> Product/1
  Kgpemf [Vs]/1 -> Product/2
  "i_GP2 [A] "/1 -> Product1/1
  Rgp [Ohm]/1 -> Product1/2
  Product1/1 -> Add/2
  Product/1 -> Add/1
  U_GP2 [V]/1 -> Add/3
  Lgp [H]/1 -> Divide/2
  Divide/1 -> Integrator/1  "di_GP2/dt [A/s]"
  Add/1 -> Divide/1
  Integrator/1 -> i_GP2 [A]/1  "i_GP2 [A]"

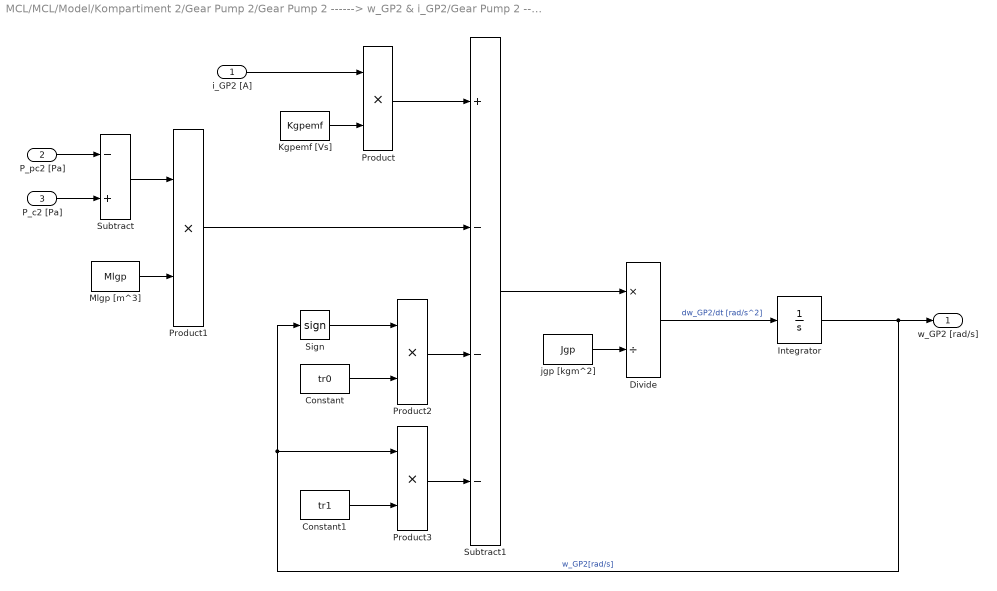
== system MCL/MCL/Model/Kompartiment 2/Gear Pump 2/Gear Pump 2 ------> w_GP2 & i_GP2/Gear Pump 2 ----> w_GP2 ==
  i_GP2 [A] : Inport
  P_pc2 [Pa] : Inport  Port=2
  P_c2 [Pa] : Inport  Port=3
  Constant : Constant  Value=tr0
  Constant1 : Constant  Value=tr1
  Divide : Product  Inputs=*/
  Integrator : Integrator
  Kgpemf [Vs] : Constant  Value=Kgpemf
  Mlgp [m^3] : Constant  Value=Mlgp
  Product{,1..3} (4 alike) : Product  RndMeth=Zero
  Sign : Signum  ZeroCross=off
  Subtract : Sum  Inputs=-+
  Subtract1 : Sum  Inputs=+---
  jgp [kgm^2] : Constant  Value=Jgp
  w_GP2 [rad/s] : Outport
  wires:
  Subtract1/1 -> Divide/1
  jgp [kgm^2]/1 -> Divide/2
  Integrator/1 -> Product3/1, Sign/1, w_GP2 [rad/s]/1  "w_GP2[rad/s]"
  Divide/1 -> Integrator/1  "dw_GP2/dt [rad/s^2]"
  i_GP2 [A]/1 -> Product/1
  Kgpemf [Vs]/1 -> Product/2
  Product/1 -> Subtract1/1
  Product1/1 -> Subtract1/2
  Subtract/1 -> Product1/1
  Mlgp [m^3]/1 -> Product1/2
  P_c2 [Pa]/1 -> Subtract/2
  P_pc2 [Pa]/1 -> Subtract/1
  Sign/1 -> Product2/1
  Constant/1 -> Product2/2
  Product3/1 -> Subtract1/4
  Constant1/1 -> Product3/2
  Product2/1 -> Subtract1/3

== matlab function MCL/Model/Kompartiment 1/VCA1/MATLAB Function ==
  data: u input double; y output double
function y = fcn(u)
%#codegen

if u>=0.0127 || u<=-0.0127
    y = 0;

else
    y=1;
end

== matlab function MCL/Model/Kompartiment 2/VCA2/MATLAB Function1 ==
  data: u input double; y output double
function y = fcn(u)
%#codegen

if u>=0.0127 || u<=-0.0127
    y = 0;

else
    y=1;
end
